simulink library "PalmaLibs"  (Simulink 8.1)
settings: Solver=ode45  SolverMode=SingleTasking  StartTime=0.0  StopTime=10.0  RelTol=1e-3
undefined symbols (not defined in the file or in its folder): gca, lambda1, lambda2, playNice, pls_solve, w_0
undefined symbols (not defined in the file): beta, w, Xpost, Xpre
libraries: simulink x9, dspmtrx3 x2, gated_decay_choice x2, range_choice x2, synaptic_scaling_choice x2, WaveformsLib x2, PalmaLibs x1, dspxfrm3 x1, CurrentsLib x1, SynapsesLib x1
settings Model: Creator=jpalma  LastModifiedBy=Leo

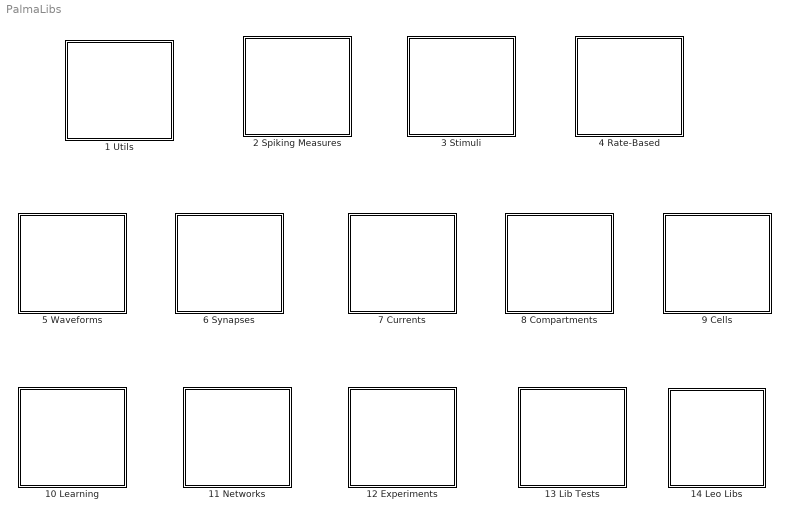
== system PalmaLibs ==
  " 1 Utils" : Subsystem
      mask help: Library Designer: Jesse Palma
      settings: OpenFcn=UtilsLib
      mask Help: Library Designer: Jesse Palma
      mask Display: image(imread('../Libs/icons/Utils.JPG'),'Center');
  " 2 Spiking Measures" : Subsystem
      mask help: Library Designer: Jesse Palma
      settings: OpenFcn=SpikingLib
      mask Help: Library Designer: Jesse Palma
      mask Display: image(imread('../Libs/icons/BasicSpike.JPG'),'Center')
  " 3 Stimuli" : Subsystem
      mask help: Library Designer: Jesse Palma
      settings: OpenFcn=StimuliLib
      mask Help: Library Designer: Jesse Palma
      mask Display: image(imread('../Libs/icons/Stimuli.JPG'),'Center')
  " 4 Rate-Based" : Subsystem
      mask help: Library Designer: Jesse Palma
      settings: OpenFcn=RateBasedLib
      mask Help: Library Designer: Jesse Palma
      mask Display: image(imread('../Libs/icons/RateBased.JPG'),'Center')
  " 5 Waveforms" : Subsystem
      mask help: Library Designer: Jesse Palma
      settings: OpenFcn=WaveformsLib
      mask Help: Library Designer: Jesse Palma
      mask Display: image(imread('../Libs/icons/DoubleExp.JPG'),'center');
  " 6 Synapses" : Subsystem
      mask help: Library Designer: Jesse Palma
      settings: OpenFcn=SynapsesLib
      mask Help: Library Designer: Jesse Palma
      mask Display: image(imread('../Libs/icons/Synapse.JPG'),'center');
  " 7 Currents" : Subsystem
      mask help: Library Designer: Jesse Palma
      settings: OpenFcn=CurrentsLib
      mask Help: Library Designer: Jesse Palma
      mask Display: image(imread('../Libs/icons/Channel.JPG'),'center');
  " 8 Compartments" : Subsystem
      mask help: Library Designer: Jesse Palma
      settings: OpenFcn=CompartmentsLib
      mask Help: Library Designer: Jesse Palma
      mask Display: image(imread('../Libs/icons/Compartment.JPG'),'Center')
  " 9 Cells" : Subsystem
      mask help: Library Designer: Jesse Palma
      settings: OpenFcn=CellsLib
      mask Help: Library Designer: Jesse Palma
      mask Display: image(imread('../Libs/icons/Cell.JPG'),'center');
  10 Learning : Subsystem
      mask help: Library Designer: Jesse Palma
      settings: OpenFcn=LearningLib
      mask Help: Library Designer: Jesse Palma
      mask Display: image(imread('../Libs/icons/Synapse.JPG'),'center');
  11 Networks : Subsystem
      mask help: Library Designer: Jesse Palma
      settings: OpenFcn=NetworksLib
      mask Help: Library Designer: Jesse Palma
      mask Display: image(imread('../Libs/icons/Networks.JPG'),'Center');
  12 Experiments : Subsystem
      mask help: Library Designer: Jesse Palma
      settings: OpenFcn=ExperimentsLib
      mask Help: Library Designer: Jesse Palma
      mask Display: image(imread('../Libs/icons/Experiments.JPG'),'Center');
  13 Lib Tests : Subsystem
      mask help: Library Designer: Jesse Palma
      settings: OpenFcn=LibTests
      mask Help: Library Designer: Jesse Palma
      mask Display: image(imread('../Libs/icons/LibTests.JPG'),'Center');
  14 Leo Libs : Subsystem

== system PalmaLibs/ 1 Utils ==

== system PalmaLibs/ 2 Spiking Measures ==

== system PalmaLibs/ 3 Stimuli ==

== system PalmaLibs/ 4 Rate-Based ==

== system PalmaLibs/ 5 Waveforms ==

== system PalmaLibs/ 6 Synapses ==

== system PalmaLibs/ 7 Currents ==

== system PalmaLibs/ 8 Compartments ==

== system PalmaLibs/ 9 Cells ==

== system PalmaLibs/10 Learning ==

== system PalmaLibs/11 Networks ==

== system PalmaLibs/12 Experiments ==

== system PalmaLibs/13 Lib Tests ==

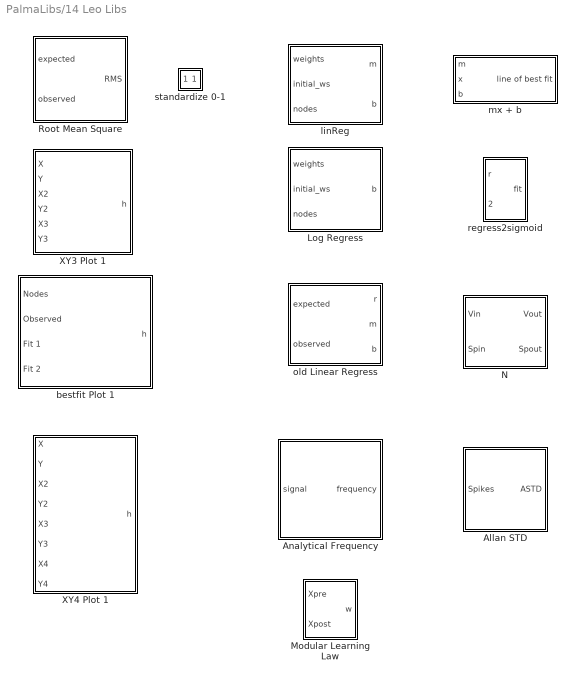
== system PalmaLibs/14 Leo Libs ==
  Allan STD : Subsystem  mask{tao=50}
      mask prompts: tao "time window"
  Analytical Frequency : Subsystem  mask{freqWindow=1}
      mask prompts: freqWindow "Window (time steps)"
      mask init:
      | freqWindow = 1;
      mask Display:
      | image(imread('../Libs/icons/hilbert.jpg'),'center');
      | port_label('input',1,'signal');
      | port_label('output',1,'freq');
  Log Regress : Subsystem  mask(Regression){numNodes=10}
      mask prompts: numNodes "Number of Nodes:"
      mask help:
      | This block does a nonlinear regression and returns the parameters necessary
      | for reconstruction
      mask init:
      | setupRegress(numNodes);
      mask Display:
      | image(imread('../Libs/icons/logfit.jpg'),'center');
      | port_label('input',1,'weights');
      | port_label('input',2,'initial weights');
      | port_label('input',3,'nodes');
      | port_label('output',1,'r');
  Modular Learning Law : Subsystem  mask{gorch_y_n=on, gated_decay=Dual OR, multdiv=Divide, synscale=Vanilla Oja, gorch_range=0, lambda1=1, lambda2=0, lambda3=0, lambda4=0, w_0=0, w0=0, alpha1=0, alpha2=0, beta=0, equ=lambda2*[Xpre*Xpost*(gorchrange)+ lambda1*(w_0-w) / ((alpha1*Xpre+alpha2*Xpost^2)*(w-w_0)) + .5lambda3*lambda4*(w_0 - w)comp(w_0,w)*(g(Xpost) - |g(Xpost)|)(g(Xpost))], extr=}
      mask prompts: gorch_y_n "Would you like a Gorch range?"; gated_decay "What kind of gated decay do you want"; multdiv "Multiply or Divide by the Gated Decay"; synscale "Synaptic Scaling"; gorch_range "Gorch Range"; lambda1 "Learning Rate (1) - Stability"; lambda2 "Learning Rate (2) - Total"; lambda3 "Learning Rate (3, Oja Specific) - Increment"; lambda4 "Learning Rate (4, Oja Specific) - Decrement"; w_0 "Range"; w0 "Initial weight"; alpha1 "Alpha 1 (Additional Parameter)"; alpha2 "Alpha 2 (Additional Parameter)"; beta "Beta (Gorch Gating Term)"; equ "Equation"; extr "Extra info"
      mask help: Make sure to hit apply after selecting your Law Type before moving on to the Law Parameters Tab.
      mask init:
      | eqw ='lambda2*[';
      | dab = gcb;
      | set_param(dab,'extr','');
      | currentVis = get_param(dab,'MaskVisibilities');
      | currentVis{12} = 'off';
      | currentVis{13} = 'off';
      | currentVis{14} = 'off';
      | 
      | if(gorch_y_n)
      |     set_param([dab '/Range'], 'BlockChoice', 'Gorch_range');
      |     currentVis{5} = 'on';
      |     eqw = [eqw 'Xpre*Xpost*(gorchrange)'];
      | else
      |     set_param([dab '/Range'], 'BlockChoice', 'Simple');
      |     currentVis{5} = 'off';
      |     eqw = [eqw 'Xpre*Xpost'];
      | end
      | 
      | eqw = [eqw '+ lambda1*(w_0-w)']
      | 
      | switch multdiv
      |     case 1 %'Multiply'
      |         set_param([dab '/TimesOrDivide'],'Inputs','**');
      |         eqw = [eqw ' * '];
      |     case 2 %'Divide'
      |         set_param([dab '/TimesOrDivide'],'Inputs','*/');
      |         eqw = [eqw ' / '];
      |     case 3 %'Inverse Divide'
      |         set_param([dab '/TimesOrDivide'],'Inputs','/*');
      |         eqw = [eqw ' \ '];
      | end
      | 
      | switch gated_decay
      |     case 1 %'Xpre'
      |         set_param([dab '/Gated Decay Choice'], 'BlockChoice', 'X_pre');
      |         eqw = [eqw 'Xpre'];
      |     case 2 %'Xpost'
      |         set_param([dab '/Gated Decay Choice'], 'BlockChoice', 'X_post');
      |         eqw = [eqw 'Xpost'];
      |     case 3 %'Gorch'
      |         set_param([dab '/Gated Decay Choice'], 'BlockChoice', 'Gorch_Gating');
      |         eqw = [eqw '(Xpost^2 * beta)'];
      |         currentVis{14} = 'on';
      |     case 4 %'Oja'
      |         set_param([dab '/Gated Decay Choice'], 'BlockChoice', 'Oja_Gating');
      |         eqw = [eqw '(Xpost^2*(w-w_0))'];
      |         currentVis{14} = 'off';
      |     case 5 %'Dual OR'
      |         set_param([dab '/Gated Decay Choice'], 'BlockChoice', 'Dual_OR');
      |         eqw = [eqw '((alpha1*Xpre+alpha2*Xpost^2)*(w-w_0))'];
      |         currentVis{12} = 'on';
      |         currentVis{13} = 'on';
      |     case 6 %'Dual AND'
      |         set_param([dab '/Gated Decay Choice'], 'BlockChoice', 'Dual_AND');
      |         eqw = [eqw '(alpha1*Xpre*Xpost^2*(w-w_0))'];
      |         currentVis{12} = 'on';
      | end
      | 
      | switch synscale
      |     case 1 %none
      |         set_param([dab '/Synaptic Scaling Choice'], 'BlockChoice', 'None');
      |         currentVis{8} = 'off';
      |         currentVis{9} = 'off';
      |         eqw = [eqw ']']
      |     case 2 %oja
      |         set_param([dab '/Synaptic Scaling Choice'], 'BlockChoice', 'Oja_stock');
      |         currentVis{8} = 'on';
      |         currentVis{9} = 'on';
      |         eqw = [eqw ' + .5lambda3*lambda4*(w_0 - w)comp(w_0,w)*(g(Xpost) - |g(Xpost)|)(g(Xpost))]'];
      |         set_param(dab,'extr','dg(X)/dt = s-AX, g(0) = -t, comp(w0,w) = |w0-w| <= range');
      | end
      | 
      | set_param(dab,'MaskVisibilities',currentVis);
      | set_param(dab,'equ',eqw);
      settings: AttributesFormatString=dw/dt = %<equ>\n%<extr>
      mask TypeOptions gated_decay: Xpre | Xpost | Gorch | Oja | Dual OR | Dual AND
      mask TypeOptions multdiv: Multiply | Divide | Inverse Divide
      mask TypeOptions synscale: None | Vanilla Oja
  N : Subsystem
  Root Mean Square : Subsystem  mask(Root Mean Square){}
      mask help: This block returns the root mean square error associated with an expected value and an observed value
      mask Display:
      | image(imread('../Libs/icons/rms.jpg'),'center');
      | port_label('input',1,'Expected');
      | port_label('input',2,'Observed');
      | port_label('output',1,'RMS');
  XY3 Plot 1 : Subsystem  AncestorBlock=UtilsLib/XY3 Plot  mask{plotInt=10, plotFig=1}
      mask prompts: plotInt "Plotting Interval (Sim steps)"; plotFig "Figure Number"
      mask help: The number of the block is the number of the figure
      mask init:
      | temp = get_param(gcb, 'Name');
      | plotFig = findLastNums(temp);
      mask Display: image(imread('../Libs/icons/XYFunc.JPG'),'center');
  XY4 Plot 1 : Subsystem  AncestorBlock=PalmaLibs/14 Leo Libs/XY3 Plot 1  mask{plotInt=10, plotFig=1}
      mask prompts: plotInt "Plotting Interval (Sim steps)"; plotFig "Figure Number"
      mask help: The number of the block is the number of the figure
      mask init:
      | temp = get_param(gcb, 'Name');
      | plotFig = findLastNums(temp);
      mask Display: image(imread('../Libs/icons/XYFunc.JPG'),'center');
  bestfit Plot 1 : Subsystem  AncestorBlock=PalmaLibs/14 Leo Libs/XY3 Plot 1  mask{plotInt=10, plotFig=1}
      mask prompts: plotInt "Plotting Interval (Sim steps)"; plotFig "Figure Number"
      mask help: The number of the block is the number of the figure
      mask init:
      | temp = get_param(gcb, 'Name');
      | plotFig = findLastNums(temp);
      mask Display: image(imread('../Libs/icons/XYFunc.JPG'),'center');
  linReg : Subsystem  mask{numNodes=10}
      mask prompts: numNodes "Number of Nodes"
      mask init:
      | setupLinRegress(numNodes)
      mask Display:
      | image(imread('../Libs/icons/regressionsweb.jpg'),'center');
      | port_label('input',1,'Weights');
      | port_label('input',2,'ws0');
      | port_label('input',3,'Nodes');
      | port_label('output',1,'m');
      | port_label('output',2,'b');
  mx + b : Subsystem
      mask help: Helper block for linReg, takes fitted params and produces the associated line
  old Linear Regress : Subsystem  mask(Regression){}
      mask help:
      | This block does a linear regression between expected and observed data in blocks of 100 trials.
      | Returns r,m,b values of regression
      mask Display:
      | image(imread('../Libs/icons/regressionsweb.jpg'),'center');
      | port_label('input',1,'Expected');
      | port_label('input',2,'Observed');
      | port_label('output',1,'r');
      | port_label('output',2,'m');
      | port_label('output',3,'b');
  regress2sigmoid : Subsystem
      mask help: Helper block for logRegress, takes fitted params and produces the associated curve
  standardize 0-1 : Subsystem
      mask help: Standardize input to range 0-1

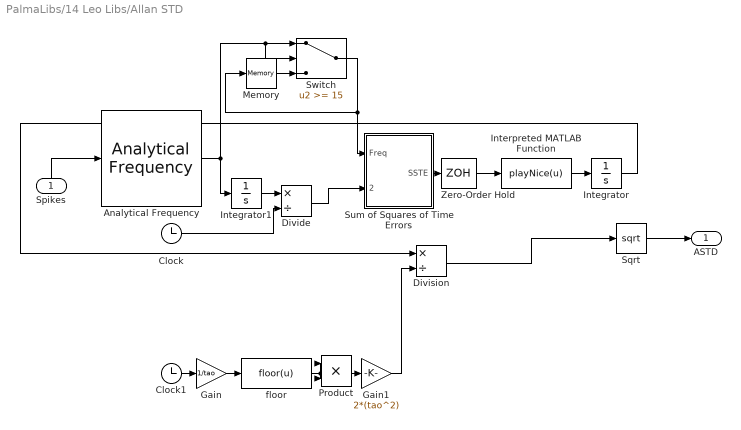
== system PalmaLibs/14 Leo Libs/Allan STD ==
  Spikes : Inport
  Analytical Frequency : PalmaLibs/14 Leo Libs/Analytical Frequency  freqWindow=1
  Clock : Clock
  Clock1 : Clock
  Divide : Product  Inputs=*/
  Division : Product  Inputs=*/
  Gain : Gain  Gain=1/tao
  Gain1 : Gain  Gain=2*(tao^2)
  Integrator : Integrator
  Integrator1 : Integrator
  Interpreted MATLAB Function : MATLABFcn  MATLABFcn=playNice(u)
  Memory : Memory
  Product : Product
  Sqrt : Sqrt  SaturateOnIntegerOverflow=on
  Sum of Squares of Time Errors : Subsystem
  Switch : Switch  Threshold=15
  Zero-Order Hold : ZeroOrderHold  SampleTime=tao
  floor : MATLABFcn  MATLABFcn=floor(u)
  ASTD : Outport
  wires:
  Sum of Squares of Time Errors/1(SSTE) -> Zero-Order Hold/1
  Clock1/1 -> Gain/1
  Gain/1 -> floor/1
  floor/1 -> Product/2, Product/1
  Product/1 -> Gain1/1
  Gain1/1 -> Division/2
  Division/1 -> Sqrt/1
  Sqrt/1 -> ASTD/1
  Integrator/1 -> Division/1
  Zero-Order Hold/1 -> Interpreted MATLAB Function/1
  Interpreted MATLAB Function/1 -> Integrator/1
  Spikes/1 -> Analytical Frequency/1
  Divide/1 -> Sum of Squares of Time Errors/2(nomFreq)
  Analytical Frequency/1 -> Switch/2, Switch/1, Integrator1/1
  Integrator1/1 -> Divide/1
  Clock/1 -> Divide/2
  Switch/1 -> Sum of Squares of Time Errors/1(Freq), Memory/1
  Memory/1 -> Switch/3

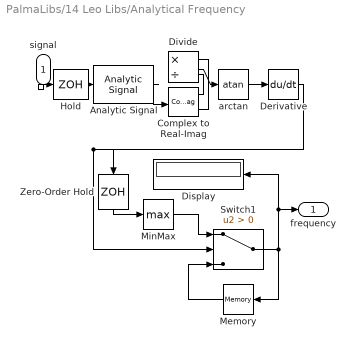
== system PalmaLibs/14 Leo Libs/Analytical Frequency ==
  signal : Inport
  Analytic Signal : dspxfrm3/Analytic Signal  N=100  InputProcessing=Columns as channels (frame based)
  Complex to Real-Imag : ComplexToRealImag
  Derivative : Derivative
  Display : Display
  Divide : Product  Inputs=*/
  Hold : ZeroOrderHold
  Memory : Memory
  MinMax : MinMax  Function=max
  Switch1 : Switch  Criteria=u2 > Threshold
  Zero-Order Hold : ZeroOrderHold  SampleTime=freqWindow
  arctan : Trigonometry  Operator=atan
  frequency : Outport
  wires:
  arctan/1 -> Derivative/1
  Divide/1 -> arctan/1
  Complex to Real-Imag/2 -> Divide/1
  Complex to Real-Imag/1 -> Divide/2
  Analytic Signal/1 -> Complex to Real-Imag/1
  Memory/1 -> Switch1/3
  Switch1/1 -> frequency/1, Display/1, Memory/1
  Zero-Order Hold/1 -> MinMax/1
  Derivative/1 -> Switch1/2, Zero-Order Hold/1
  MinMax/1 -> Switch1/1
  signal/1 -> Hold/1
  Hold/1 -> Analytic Signal/1

== system PalmaLibs/14 Leo Libs/Log Regress ==
  weights : Inport
  initial_ws : Inport  Port=2
  nodes : Inport  Port=3
  Compare To Constant : simulink/Logic and Bit Operations/Compare To Constant  relop=<=  const=Inf  OutDataTypeStr=uint8
  Hold1 : ZeroOrderHold  SampleTime=100
  Hold2 : ZeroOrderHold  SampleTime=100
  Hold3 : ZeroOrderHold  SampleTime=100
  Switch : Switch  Threshold=1
  Transpose : dspmtrx3/Transpose  Hermitian=off  overflowFlag=off
  Vector Concatenate : Concatenate
  solver : MATLABFcn  MATLABFcn=pls_solve([u(11),u(12),u(13),u(14),u(15),u(16),u(17),u(18),u(19),u(20)],[u(1),u(2),u(3),u(4),u(5),u(6),u(7),u(8),u(9),u(10)],[ 0.1 0 0.1])
  b : Outport
  wires:
  Hold3/1 -> Vector Concatenate/2
  Hold2/1 -> Switch/3
  Vector Concatenate/1 -> solver/1
  nodes/1 -> Hold3/1
  initial_ws/1 -> Hold2/1
  Switch/1 -> Vector Concatenate/1
  Compare To Constant/1 -> Switch/2
  Transpose/1 -> Switch/1, Compare To Constant/1
  Hold1/1 -> Transpose/1
  weights/1 -> Hold1/1
  solver/1 -> b/1

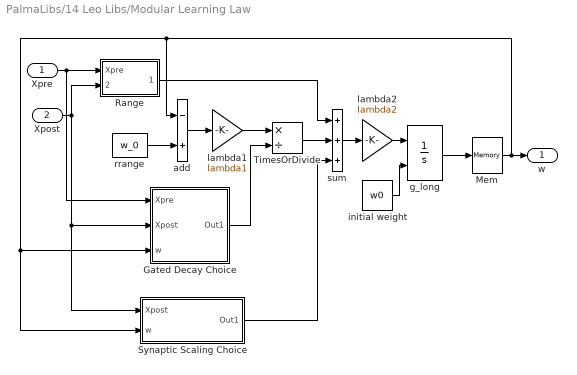
== system PalmaLibs/14 Leo Libs/Modular Learning Law ==
  Xpre : Inport
  Xpost : Inport  Port=2
  Gated Decay Choice : Subsystem  BlockChoice=Dual_OR
      settings: AttributesFormatString=%<BlockChoice>  TemplateBlock=gated_decay_choice/Gated Decay Choice  MemberBlocks=Dual_AND,Dual_OR,Gorch_Gating,Oja_Gating,X_post,X_pre
  Mem : Memory
  Range : Subsystem  BlockChoice=Gorch_range
      link override Gorch_range/range: Value=gorch_range
      settings: AttributesFormatString=%<BlockChoice>  TemplateBlock=range_choice/Range  MemberBlocks=Gorch_range,Simple
  Synaptic Scaling Choice : Subsystem  BlockChoice=Oja_stock
      settings: AttributesFormatString=%<BlockChoice>  TemplateBlock=synaptic_scaling_choice/Synaptic Scaling Choice  MemberBlocks=None,Oja_stock
  TimesOrDivide : Product  Inputs=*/
  add : Sum  Inputs=-+
  g_long : Integrator  InitialConditionSource=external  ZeroCross=off
  initial weight : Constant  Value=w0
  lambda1 : Gain  Gain=lambda1
  lambda2 : Gain  Gain=lambda2
  rrange : Constant  Value=w_0
  sum : Sum  Inputs=+++
  w : Outport
  wires:
  Xpre/1 -> Range/1(Xpre), Gated Decay Choice/1(Xpre)
  Xpost/1 -> Gated Decay Choice/2(Xpost), Synaptic Scaling Choice/1(Xpost), Range/2(Xpost)
  rrange/1 -> add/2
  Range/1(Out1) -> sum/1
  add/1 -> lambda1/1
  lambda1/1 -> TimesOrDivide/1
  TimesOrDivide/1 -> sum/2
  g_long/1 -> Mem/1
  initial weight/1 -> g_long/2
  Mem/1 -> Synaptic Scaling Choice/2(w), Gated Decay Choice/3(w), add/1, w/1
  Gated Decay Choice/1(Out1) -> TimesOrDivide/2
  lambda2/1 -> g_long/1
  sum/1 -> lambda2/1
  Synaptic Scaling Choice/1(Out1) -> sum/3

== system PalmaLibs/14 Leo Libs/N ==
  Vin : Inport
  Spin : Inport  Port=2
  AMPASynapse : Subsystem  AncestorBlock=SynapsesLib/CompoundDiffSynapse  mask{EZ=0, gZ=0.05, tauRZ=1, tauFZ=6}
      mask prompts: EZ "Eq Voltage, EZ"; gZ "Conductance, gZ"; tauRZ "Rise Time, tauRZ"; tauFZ "Fall Time, tauFZ"
      mask help: Author: Jesse Palma
      mask Help: Author: Jesse Palma
      mask Display: image(imread('../Libs/icons/Synapse.jpg'),'center');
  Add : Sum
  Izhikevich Book1 : Subsystem  AncestorBlock=CompartmentsLib/Izhikevich Book  mask{settings=UserDefined, A=0.03, B=-2, C=-50, D=100, CP=100, K=0.7, VR=-60, VT=-40, VP=35, V0=-60, U0=0}
      mask prompts: settings "Parameter Settings"; A "a, recovery u time constant"; B "b, dynamics parameter"; C "c,  reset value v"; D "d, reset shift u"; CP "Cp, capacitance"; VR "Vr, voltage rest"; VT "Vt, voltage threshold"; VP "Vpeak, voltage peak reset"; V0 "V0, initial v value"; U0 "U0, initial u value"
      mask help:
      | Model from Eugene Izhikevich's book "Dynamical Systems in Neuroscience"
      |     (Equations 8.5 & 8.6 on page 273)
      | 9 Paramters are reducable to 4-parameter model.
      |
      | Simulink Model Design: Jesse Palma
      mask Help:
      | Model from Eugene Izhikevich's book
      | <a href=http://www.izhikevich.org/publications/dsn/index.htm>"Dynamical Systems in Neuroscience"</a>
      | <br>(Equations 8.5 & 8.6 on page 273)<br>
      | 9 Paramters are reducable to 4-parameter model.
      | <br><br>
      | Simulink Model Design: Jesse Palma
      mask TypeOptions settings: Regular-Spiking(p274-283) | Motor(p287) | UserDefined
      mask Callback settings:
      | maskStr = get_param(gcb,'MaskValues');
      | if strcmp(maskStr{1},'Regular-Spiking(p274-283)')
      |    maskStr = get_param(gcb,'MaskValues');
      |    maskStr{2} = '0.03'; %A
      |    maskStr{3} = '-2';   %B
      |    maskStr{4} = '-50';  %C
      |    maskStr{5} = '100';  %D
      |    maskStr{6} = '100';  %CP
      |    maskStr{7} = '0.7';  %K
      |    maskStr{8} = '-60';  %VR
      |    maskStr{9} = '-40';  %VT
      |    maskStr{10} = '35';  %VP
      |    maskStr{11} = '-60'; %V0
      |    maskStr{12} = '0';   %U0
      |    set_param(gcb, 'MaskValues', maskStr);
      | end
      | if strcmp(maskStr{1},'Motor(p287)')
      |    maskStr = get_param(gcb,'MaskValues');
      |    maskStr{2} = '0.01'; %A
      |    maskStr{3} = '-0.25';%B
      |    maskStr{4} = '-40';  %C
      |    maskStr{5} = '90';   %D
      |    maskStr{6} = '30';   %CP
      |    maskStr{7} = '3';    %K
      |    maskStr{8} = '-55';  %VR
      |    maskStr{9} = '-42';  %VT
      |    maskStr{10} = '10';  %VP
      |    maskStr{11} = '-55'; %V0
      |    maskStr{12} = '0';   %U0
      |    set_param(gcb, 'MaskValues', maskStr);
      | end
      mask Callback A:
      | maskStr = get_param(gcb,'MaskValues');
      | maskStr{1} = 'UserDefined';
      | set_param(gcb, 'MaskValues', maskStr);
      mask Callback B:
      | maskStr = get_param(gcb,'MaskValues');
      | maskStr{1} = 'UserDefined';
      | set_param(gcb, 'MaskValues', maskStr);
      mask Callback C:
      | maskStr = get_param(gcb,'MaskValues');
      | maskStr{1} = 'UserDefined';
      | set_param(gcb, 'MaskValues', maskStr);
      mask Callback D:
      | maskStr = get_param(gcb,'MaskValues');
      | maskStr{1} = 'UserDefined';
      | set_param(gcb, 'MaskValues', maskStr);
      mask Callback CP:
      | maskStr = get_param(gcb,'MaskValues');
      | maskStr{1} = 'UserDefined';
      | set_param(gcb, 'MaskValues', maskStr);
      mask Callback K:
      | maskStr = get_param(gcb,'MaskValues');
      | maskStr{1} = 'UserDefined';
      | set_param(gcb, 'MaskValues', maskStr);
      mask Callback VR:
      | maskStr = get_param(gcb,'MaskValues');
      | maskStr{1} = 'UserDefined';
      | set_param(gcb, 'MaskValues', maskStr);
      mask Callback VT:
      | maskStr = get_param(gcb,'MaskValues');
      | maskStr{1} = 'UserDefined';
      | set_param(gcb, 'MaskValues', maskStr);
      mask Callback VP:
      | maskStr = get_param(gcb,'MaskValues');
      | maskStr{1} = 'UserDefined';
      | set_param(gcb, 'MaskValues', maskStr);
      mask Callback V0:
      | maskStr = get_param(gcb,'MaskValues');
      | maskStr{1} = 'UserDefined';
      | set_param(gcb, 'MaskValues', maskStr);
      mask Callback U0:
      | maskStr = get_param(gcb,'MaskValues');
      | maskStr{1} = 'UserDefined';
      | set_param(gcb, 'MaskValues', maskStr);
      mask Display: image(imread('../Libs/icons/Izhik.jpg'),'center');
  Learning Law : Subsystem  mask{gorch_y_n=off, gated_decay=Gorch, multdiv=Multiply, synscale=None, gorch_range=0, lambda1=.05, lambda2=.05, lambda3=0, lambda4=0, w_0=1, w0=.3, beta=1, equ=lambda2*[Xpre*Xpost+ lambda1*(w_0-w) * (Xpost^2 * beta)], extr=}
      mask prompts: gorch_y_n "Would you like a Gorch range?"; gated_decay "What kind of gated decay do you want"; multdiv "Multiply or Divide by the Gated Decay"; synscale "Synaptic Scaling"; gorch_range "Gorch Range"; lambda1 "Learning Rate (1) - Stability"; lambda2 "Learning Rate (2) - Total"; lambda3 "Learning Rate (3, Oja Specific) - Increment"; lambda4 "Learning Rate (4, Oja Specific) - Decrement"; w_0 "Range"; w0 "Initial weight"; beta "Beta (Gorch Gating Term)"; equ "Equation"; extr "Extra info"
      mask help: Make sure to hit apply after selecting your Law Type before moving on to the Law Parameters Tab.
      mask init:
      | eqw ='lambda2*[';
      | dab = gcb;
      | set_param(dab,'extr','');
      | currentVis = get_param(dab,'MaskVisibilities');
      | if(gorch_y_n)
      |     set_param([dab '/Range'], 'BlockChoice', 'Gorch_range');
      |     currentVis{5} = 'on';
      |     eqw = [eqw 'Xpre*Xpost*(gorchrange)'];
      | else
      |     set_param([dab '/Range'], 'BlockChoice', 'Simple');
      |     currentVis{5} = 'off';
      |     currentVis{12} = 'off';
      |     eqw = [eqw 'Xpre*Xpost'];
      | end
      | eqw = [eqw '+ lambda1*(w_0-w)']
      | switch multdiv
      |     case 1 %'Multiply'
      |         set_param([dab '/TimesOrDivide'],'Inputs','**');
      |         eqw = [eqw ' * '];
      |     case 2 %'Divide'
      |         set_param([dab '/TimesOrDivide'],'Inputs','*/');
      |         eqw = [eqw ' / '];
      |         
      |     case 3 %'Inverse Divide'
      |         set_param([dab '/TimesOrDivide'],'Inputs','/*');
      |         eqw = [eqw ' \ '];
      |         
      | end
      | switch gated_decay
      |     case 1 %'Xpre'
      |         set_param([dab '/Gated Decay Choice'], 'BlockChoice', 'X_pre');
      |         eqw = [eqw 'Xpre'];
      |         currentVis{12} = 'off';
      |         
      |     case 2 %'Xpost'
      |         set_param([dab '/Gated Decay Choice'], 'BlockChoice', 'X_post');
      |         eqw = [eqw 'Xpost'];
      |         currentVis{12} = 'off';
      |         
      |     case 3 %'Gorch'
      |         set_param([dab '/Gated Decay Choice'], 'BlockChoice', 'Gorch_Gating');
      |         eqw = [eqw '(Xpost^2 * beta)'];
      |         currentVis{12} = 'on';
      |         
      |     case 4 %'Oja'
      |         set_param([dab '/Gated Decay Choice'], 'BlockChoice', 'Oja_Gating');
      |         eqw = [eqw '(Xpost^2*(w-w_0))'];
      |         currentVis{12} = 'off';
      |         
      | end
      | 
      | switch synscale
      |     case 1 %none
      |         set_param([dab '/Synaptic Scaling Choice'], 'BlockChoice', 'None');
      |         currentVis{8} = 'off';
      |         currentVis{9} = 'off';
      |         eqw = [eqw ']']
      |     case 2 %oja
      |         set_param([dab '/Synaptic Scaling Choice'], 'BlockChoice', 'Oja_stock');
      |         currentVis{8} = 'on';
      |         currentVis{9} = 'on';
      |         eqw = [eqw ' + .5lambda3*lambda4*(w_0 - w)comp(w_0,w)*(g(Xpost) - |g(Xpost)|)(g(Xpost))]'];
      |         set_param(dab,'extr','dg(X)/dt = s-AX, g(0) = -t, comp(w0,w) = |w0-w| <= range');
      | end
      | set_param(dab,'MaskVisibilities',currentVis);
      | set_param(dab,'equ',eqw);
      settings: AttributesFormatString=dw/dt = %<equ>\n%<extr>
      mask TypeOptions gated_decay: Xpre | Xpost | Gorch | Oja
      mask TypeOptions multdiv: Multiply | Divide | Inverse Divide
      mask TypeOptions synscale: None | Vanilla Oja
  Memory : Memory  X0=0.3
  NMDASynapse1 : SynapsesLib/NMDASynapse  EZ=0  gZ=0.005  tauRZ=0.33  tauFZ=40  etaZ=0.33  mgZ=1  gammaZ=0.06  gainZ=4
  Spike Simpl : WaveformsLib/Spike Simpl  a=-0.2  b=0.65  c=0.05
  gain1 : Gain  Gain=45
  Vout : Outport
  Spout : Outport  Port=2
  wires:
  Spin/1 -> Learning Law/1(Xpre), NMDASynapse1/1, AMPASynapse/1(spike_i)
  Vin/1 -> AMPASynapse/3(postv_j), NMDASynapse1/3
  gain1/1 -> Izhikevich Book1/1(I)
  Add/1 -> gain1/1
  NMDASynapse1/3 -> Add/1
  AMPASynapse/3(I) -> Add/2
  Izhikevich Book1/3(sp) -> Spike Simpl/2
  Izhikevich Book1/1(v) -> Vout/1, Spike Simpl/1
  Spike Simpl/1 -> Learning Law/2(Xpost), Spout/1
  Learning Law/1(w) -> Memory/1
  Memory/1 -> NMDASynapse1/2, AMPASynapse/2(w_ij)

== system PalmaLibs/14 Leo Libs/Root Mean Square ==
  expected : Inport
  observed : Inport  Port=2
  Gain : Gain  Gain=.5
  Hold : ZeroOrderHold  SampleTime=100
  Hold1 : ZeroOrderHold  SampleTime=100
  Sqrt : Sqrt  SaturateOnIntegerOverflow=on
  Sum : Sum  Inputs=|+-
  square : Math  Operator=square  SaturateOnIntegerOverflow=on
  RMS : Outport
  wires:
  expected/1 -> Hold/1
  observed/1 -> Hold1/1
  Hold1/1 -> Sum/2
  Hold/1 -> Sum/1
  Sum/1 -> square/1
  Gain/1 -> Sqrt/1
  Sqrt/1 -> RMS/1
  square/1 -> Gain/1

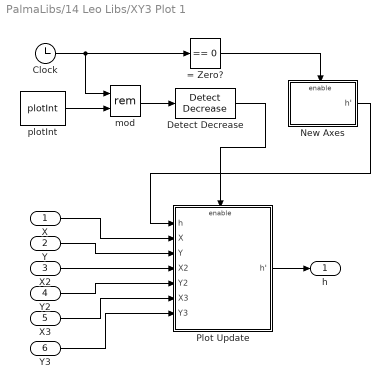
== system PalmaLibs/14 Leo Libs/XY3 Plot 1 ==
  X : Inport
  Y : Inport  Port=2
  X2 : Inport  Port=3
  Y2 : Inport  Port=4
  X3 : Inport  Port=5
  Y3 : Inport  Port=6
  = Zero? : simulink/Logic and Bit Operations/Compare To Zero  relop===  OutDataTypeStr=uint8
  Clock : Clock
  Detect Decrease : simulink/Logic and Bit Operations/Detect Decrease  vinit=0.0  InputProcessing=Inherited  OutDataTypeStr=uint8
  New Axes : Subsystem
  Plot Update : Subsystem
  mod : Math  Operator=rem  SaturateOnIntegerOverflow=on
  plotInt : Constant  Value=plotInt
  h : Outport
  wires:
  Y2/1 -> Plot Update/5(Y2)
  X2/1 -> Plot Update/4(X2)
  X/1 -> Plot Update/2(X)
  Plot Update/1(h') -> h/1
  Y/1 -> Plot Update/3(Y)
  plotInt/1 -> mod/2
  Clock/1 -> mod/1, = Zero?/1
  mod/1 -> Detect Decrease/1
  = Zero?/1 -> New Axes/Enable
  Detect Decrease/1 -> Plot Update/Enable
  New Axes/1(h') -> Plot Update/1(h)
  X3/1 -> Plot Update/6(X3)
  Y3/1 -> Plot Update/7(Y3)

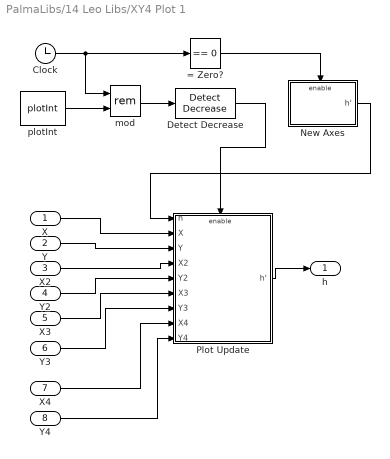
== system PalmaLibs/14 Leo Libs/XY4 Plot 1 ==
  X : Inport
  Y : Inport  Port=2
  X2 : Inport  Port=3
  Y2 : Inport  Port=4
  X3 : Inport  Port=5
  Y3 : Inport  Port=6
  X4 : Inport  Port=7
  Y4 : Inport  Port=8
  = Zero? : simulink/Logic and Bit Operations/Compare To Zero  relop===  OutDataTypeStr=uint8
  Clock : Clock
  Detect Decrease : simulink/Logic and Bit Operations/Detect Decrease  vinit=0.0  InputProcessing=Inherited  OutDataTypeStr=uint8
  New Axes : Subsystem
  Plot Update : Subsystem
  mod : Math  Operator=rem  SaturateOnIntegerOverflow=on
  plotInt : Constant  Value=plotInt
  h : Outport
  wires:
  Y3/1 -> Plot Update/7(Y3)
  X3/1 -> Plot Update/6(X3)
  New Axes/1(h') -> Plot Update/1(h)
  Detect Decrease/1 -> Plot Update/Enable
  = Zero?/1 -> New Axes/Enable
  mod/1 -> Detect Decrease/1
  Clock/1 -> = Zero?/1, mod/1
  plotInt/1 -> mod/2
  Y/1 -> Plot Update/3(Y)
  Plot Update/1(h') -> h/1
  X/1 -> Plot Update/2(X)
  X2/1 -> Plot Update/4(X2)
  Y2/1 -> Plot Update/5(Y2)
  X4/1 -> Plot Update/8(X4)
  Y4/1 -> Plot Update/9(Y4)

== system PalmaLibs/14 Leo Libs/bestfit Plot 1 ==
  Nodes : Inport
  Observed : Inport  Port=2
  Fit 1 : Inport  Port=3
  Fit 2 : Inport  Port=4
  = Zero? : simulink/Logic and Bit Operations/Compare To Zero  relop===  OutDataTypeStr=uint8
  Clock : Clock
  Detect Decrease : simulink/Logic and Bit Operations/Detect Decrease  vinit=0.0  InputProcessing=Inherited  OutDataTypeStr=uint8
  New Axes : Subsystem
  Plot Update : Subsystem
  mod : Math  Operator=rem  SaturateOnIntegerOverflow=on
  plotInt : Constant  Value=plotInt
  h : Outport
  wires:
  Fit 1/1 -> Plot Update/5(Y2)
  Nodes/1 -> Plot Update/2(X), Plot Update/4(X2), Plot Update/6(X3)
  Plot Update/1(h') -> h/1
  Observed/1 -> Plot Update/3(Y)
  plotInt/1 -> mod/2
  Clock/1 -> mod/1, = Zero?/1
  mod/1 -> Detect Decrease/1
  = Zero?/1 -> New Axes/Enable
  Detect Decrease/1 -> Plot Update/Enable
  New Axes/1(h') -> Plot Update/1(h)
  Fit 2/1 -> Plot Update/7(Y3)

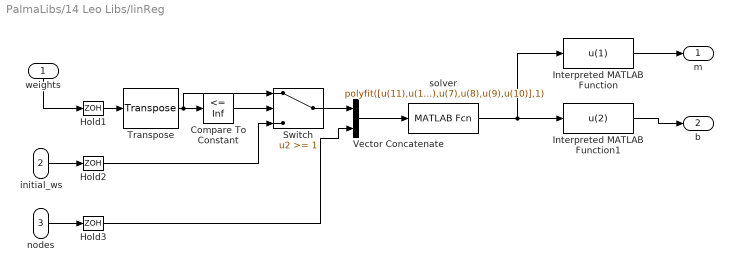
== system PalmaLibs/14 Leo Libs/linReg ==
  weights : Inport
  initial_ws : Inport  Port=2
  nodes : Inport  Port=3
  Compare To Constant : simulink/Logic and Bit Operations/Compare To Constant  relop=<=  const=Inf  OutDataTypeStr=uint8
  Hold1 : ZeroOrderHold  SampleTime=100
  Hold2 : ZeroOrderHold  SampleTime=100
  Hold3 : ZeroOrderHold  SampleTime=100
  Interpreted MATLAB Function : MATLABFcn  MATLABFcn=u(1)
  Interpreted MATLAB Function1 : MATLABFcn  MATLABFcn=u(2)
  Switch : Switch  Threshold=1
  Transpose : dspmtrx3/Transpose  Hermitian=off  overflowFlag=off
  Vector Concatenate : Concatenate
  solver : MATLABFcn  MATLABFcn=polyfit([u(11),u(12),u(13),u(14),u(15),u(16),u(17),u(18),u(19),u(20)],[u(1),u(2),u(3),u(4),u(5),u(6),u(7),u(8),u(9),u(10)],1)  mask{numNodes=0}
      mask prompts: numNodes "Number of Nodes"
      mask init:
      | %setupLinRegress(numNodes);
  m : Outport
  b : Outport  Port=2
  wires:
  Hold2/1 -> Switch/3
  Hold3/1 -> Vector Concatenate/2
  Hold1/1 -> Transpose/1
  Vector Concatenate/1 -> solver/1
  weights/1 -> Hold1/1
  Transpose/1 -> Compare To Constant/1, Switch/1
  Compare To Constant/1 -> Switch/2
  Switch/1 -> Vector Concatenate/1
  initial_ws/1 -> Hold2/1
  nodes/1 -> Hold3/1
  solver/1 -> Interpreted MATLAB Function/1, Interpreted MATLAB Function1/1
  Interpreted MATLAB Function/1 -> m/1
  Interpreted MATLAB Function1/1 -> b/1

== system PalmaLibs/14 Leo Libs/mx + b ==
  note: mx + b
  m : Inport
  x : Inport  Port=2
  b : Inport  Port=3
  Product1 : Product  RndMeth=Zero
  Sum1 : Sum  Inputs=|++
  line of best fit : Outport
  wires:
  Product1/1 -> Sum1/1
  Sum1/1 -> line of best fit/1
  m/1 -> Product1/1
  x/1 -> Product1/2
  b/1 -> Sum1/2

== system PalmaLibs/14 Leo Libs/old Linear Regress ==
  expected : Inport
  observed : Inport  Port=2
  Hold : ZeroOrderHold  SampleTime=100
  Hold1 : ZeroOrderHold  SampleTime=100
  regress b : M-S-Function  FunctionName=regress_block3
  regress m : M-S-Function  FunctionName=regress_block2
  regress r : M-S-Function  FunctionName=regress_block
  r : Outport
  m : Outport  Port=2
  b : Outport  Port=3
  wires:
  regress r/1 -> r/1
  regress m/1 -> m/1
  regress b/1 -> b/1
  observed/1 -> Hold1/1
  Hold1/1 -> regress r/2, regress m/2, regress b/2
  expected/1 -> Hold/1
  Hold/1 -> regress r/1, regress m/1, regress b/1

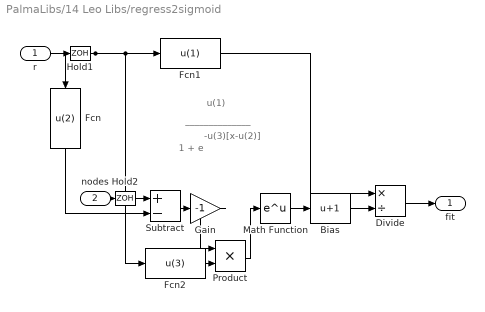
== system PalmaLibs/14 Leo Libs/regress2sigmoid ==
  note: ______________
  note: u(1)
  note: 1 + e
  note: -u(3)[x-u(2)]
  r : Inport
  nodes : Inport  Port=2
  Bias : Bias  Bias=1
  Divide : Product  Inputs=*/
  Fcn : Fcn  Expr=u(2)
  Fcn1 : Fcn  Expr=u(1)
  Fcn2 : Fcn  Expr=u(3)
  Gain : Gain  Gain=-1
  Hold1 : ZeroOrderHold  SampleTime=100
  Hold2 : ZeroOrderHold  SampleTime=100
  Math Function : Math  SaturateOnIntegerOverflow=on
  Product : Product  RndMeth=Zero
  Subtract : Sum  Inputs=+-
  fit : Outport
  wires:
  r/1 -> Hold1/1
  Fcn1/1 -> Divide/1
  Fcn/1 -> Subtract/2
  Math Function/1 -> Bias/1
  Bias/1 -> Divide/2
  nodes/1 -> Hold2/1
  Subtract/1 -> Gain/1
  Gain/1 -> Product/1
  Divide/1 -> fit/1
  Hold1/1 -> Fcn1/1, Fcn2/1, Fcn/1
  Hold2/1 -> Subtract/1
  Fcn2/1 -> Product/2
  Product/1 -> Math Function/1

== system PalmaLibs/14 Leo Libs/standardize 0-1 ==
  note: input will be time saturated data,
      | so i'll only normalize however much
      | there is for a certain interval for the
      | regression to work through
  note: Standardize X to range 0-1:
  Xi : Inport
  Divide : Product  Inputs=*/
  MinMax : MinMax
  MinMax1 : MinMax  Function=max
  Subtract : Sum  Inputs=+-
  Subtract1 : Sum  Inputs=-+
  Zero-Order Hold : ZeroOrderHold  SampleTime=100
  Si : Outport
  wires:
  Xi/1 -> Zero-Order Hold/1, Subtract/1
  Zero-Order Hold/1 -> MinMax/1, MinMax1/1
  Subtract/1 -> Divide/1
  Divide/1 -> Si/1
  MinMax/1 -> Subtract/2, Subtract1/1
  MinMax1/1 -> Subtract1/2
  Subtract1/1 -> Divide/2

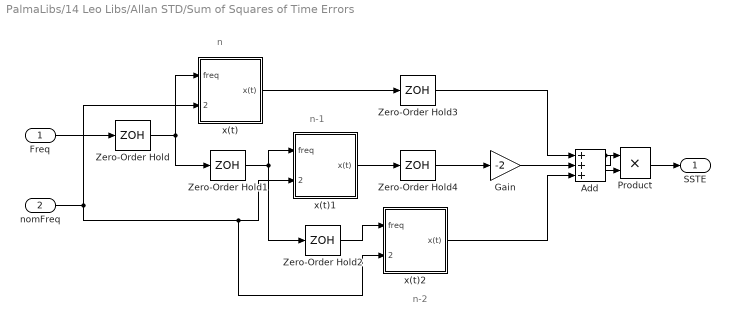
== system PalmaLibs/14 Leo Libs/Allan STD/Sum of Squares of Time Errors ==
  note: n
  note: n-2
  note: n-1
  Freq : Inport
  nomFreq : Inport  Port=2
  Add : Sum  Inputs=+++
  Gain : Gain  Gain=-2
  Product : Product
  Zero-Order Hold{,1..2,4} (4 alike) : ZeroOrderHold  SampleTime=tao
  Zero-Order Hold3 : ZeroOrderHold  SampleTime=2*tao
  x(t) : Subsystem
  x(t)1 : Subsystem
  x(t)2 : Subsystem
  SSTE : Outport
  wires:
  Gain/1 -> Add/2
  x(t)2/1(x(t)) -> Add/3
  Zero-Order Hold3/1 -> Add/1
  Zero-Order Hold4/1 -> Gain/1
  Add/1 -> Product/2, Product/1
  Zero-Order Hold1/1 -> x(t)1/1(freq), Zero-Order Hold2/1
  Zero-Order Hold/1 -> Zero-Order Hold1/1, x(t)/1(freq)
  x(t)/1(x(t)) -> Zero-Order Hold3/1
  x(t)1/1(x(t)) -> Zero-Order Hold4/1
  Zero-Order Hold2/1 -> x(t)2/1(freq)
  Freq/1 -> Zero-Order Hold/1
  Product/1 -> SSTE/1
  nomFreq/1 -> x(t)/2(nom_freq), x(t)2/2(nom_freq), x(t)1/2(nom_freq)

== system PalmaLibs/14 Leo Libs/Modular Learning Law/Gated Decay Choice ==
  Xpre : Inport
  Xpost : Inport  Port=2
  w : Inport  Port=3
  Dual_OR : gated_decay_choice/Dual_OR
  Out1 : Outport
  wires:
  Xpre/1 -> Dual_OR/1
  Xpost/1 -> Dual_OR/2
  w/1 -> Dual_OR/3
  Dual_OR/1 -> Out1/1

== system PalmaLibs/14 Leo Libs/Modular Learning Law/Range ==
  Xpre : Inport
  Xpost : Inport  Port=2
  Gorch_range : range_choice/Gorch_range
  Out1 : Outport
  wires:
  Xpre/1 -> Gorch_range/1
  Xpost/1 -> Gorch_range/2
  Gorch_range/1 -> Out1/1

== system PalmaLibs/14 Leo Libs/Modular Learning Law/Synaptic Scaling Choice ==
  Xpost : Inport
  w : Inport  Port=2
  Oja_stock : synaptic_scaling_choice/Oja_stock
  Out1 : Outport
  wires:
  Xpost/1 -> Oja_stock/1
  w/1 -> Oja_stock/2
  Oja_stock/1 -> Out1/1

== system PalmaLibs/14 Leo Libs/N/AMPASynapse ==
  spike_i : Inport
  w_ij : Inport  Port=2
  postv_j : Inport  Port=3
  Compound Diffentials : WaveformsLib/Compound Diffentials  tauRise=tauRZ  tauFall=tauFZ  squareWaveWidth=tauRZ  squareWaveHeight=1/tauRZ  interGain=2/tauRZ  finalGain=(tauFZ+tauRZ)/tauFZ
  Product : Product  RndMeth=Zero
  Sum_i : Product  Multiplication=Matrix(*)
  Ungated Current : CurrentsLib/Ungated Current  EX=EZ  gX=gZ
  T : Outport
  g : Outport  Port=2
  I : Outport  Port=3
  wires:
  w_ij/1 -> Sum_i/1
  Compound Diffentials/2 -> Sum_i/2
  Sum_i/1 -> g/1, Product/1
  postv_j/1 -> Ungated Current/1
  Compound Diffentials/1 -> T/1
  Ungated Current/1 -> Product/2
  spike_i/1 -> Compound Diffentials/1
  Product/1 -> I/1

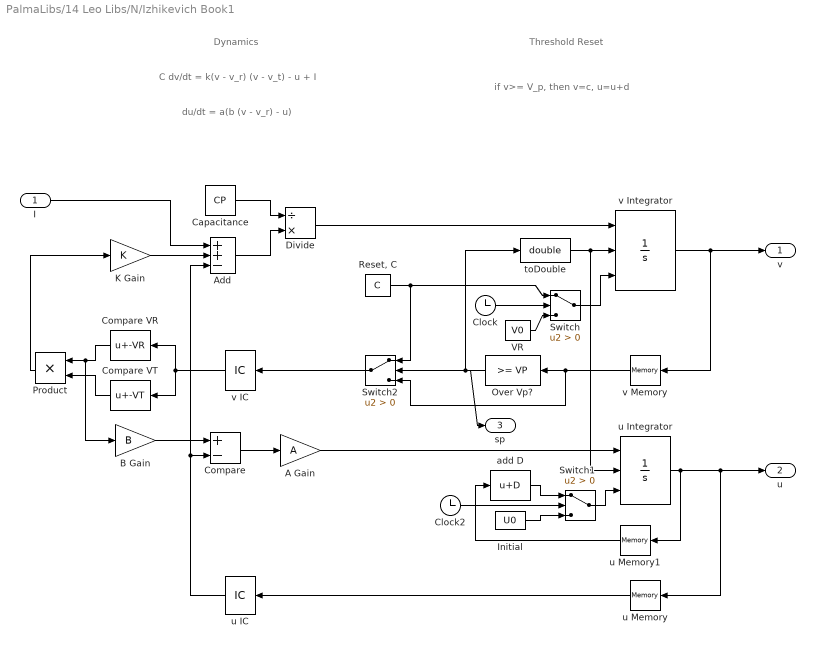
== system PalmaLibs/14 Leo Libs/N/Izhikevich Book1 ==
  note: C dv/dt = k(v - v_r) (v - v_t) - u + I
  note: du/dt = a(b (v - v_r) - u)
  note: if v>= V_p, then
      | v=c, u=u+d
  note: Dynamics
  note: Threshold Reset
  I : Inport
  " Initial" : Constant  Value=U0
  A Gain : Gain  Gain=A
  Add : Sum  Inputs=++-
  B Gain : Gain  Gain=B
  Capacitance : Constant  Value=CP
  Clock : Clock
  Clock2 : Clock
  Compare : Sum  Inputs=+-
  Compare VR : Bias  Bias=-VR
  Compare VT : Bias  Bias=-VT
  Divide : Product  Inputs=/*
  K Gain : Gain  Gain=K
  Over Vp? : simulink/Logic and Bit Operations/Compare To Constant  relop=>=  const=VP  OutDataTypeStr=boolean  ZeroCross=off
  Product : Product  RndMeth=Zero
  "Reset, C" : Constant  Value=C
  Switch : Switch  Criteria=u2 > Threshold  ZeroCross=off
  Switch1 : Switch  Criteria=u2 > Threshold  ZeroCross=off
  Switch2 : Switch  Criteria=u2 > Threshold  ZeroCross=off
  VR : Constant  Value=V0
  add D : Bias  Bias=D
  toDouble : DataTypeConversion  OutDataTypeStr=double
  u IC : InitialCondition  Value=U0
  u Integrator : Integrator  ExternalReset=rising  InitialConditionSource=external  ZeroCross=off
  u Memory : Memory
  u Memory1 : Memory
  v IC : InitialCondition  Value=V0
  v Integrator : Integrator  ExternalReset=rising  InitialConditionSource=external  InitialCondition=VR  ZeroCross=off
  v Memory : Memory
  v : Outport
  u : Outport  Port=2
  sp : Outport  Port=3
  wires:
  u Memory1/1 -> add D/1
  VR/1 -> Switch/3
  Capacitance/1 -> Divide/1
  Add/1 -> Divide/2
  toDouble/1 -> v Integrator/2, u Integrator/2
  v Integrator/1 -> v/1, v Memory/1
  K Gain/1 -> Add/2
  Compare VT/1 -> Product/2
  Compare VR/1 -> B Gain/1, Product/1
  I/1 -> Add/1
  Product/1 -> K Gain/1
  u Memory/1 -> u IC/1
  B Gain/1 -> Compare/1
  Compare/1 -> A Gain/1
  v IC/1 -> Compare VT/1, Compare VR/1
  u IC/1 -> Add/3, Compare/2
  Switch/1 -> v Integrator/3
  Clock/1 -> Switch/2
  "Reset, C"/1 -> Switch2/1, Switch/1
  u Integrator/1 -> u Memory1/1, u/1, u Memory/1
  Divide/1 -> v Integrator/1
  A Gain/1 -> u Integrator/1
  Clock2/1 -> Switch1/2
  Switch1/1 -> u Integrator/3
  add D/1 -> Switch1/1
  " Initial"/1 -> Switch1/3
  Switch2/1 -> v IC/1
  v Memory/1 -> Switch2/3, Over Vp?/1
  Over Vp?/1 -> sp/1, Switch2/2, toDouble/1

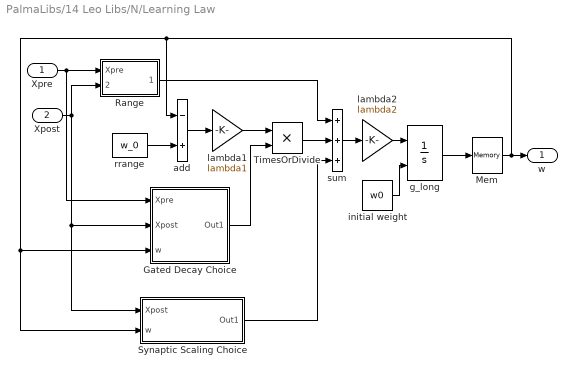
== system PalmaLibs/14 Leo Libs/N/Learning Law ==
  Xpre : Inport
  Xpost : Inport  Port=2
  Gated Decay Choice : Subsystem  BlockChoice=Gorch_Gating
      settings: AttributesFormatString=%<BlockChoice>  TemplateBlock=gated_decay_choice/Gated Decay Choice  MemberBlocks=Gorch_Gating,Oja_Gating,X_post,X_pre
  Mem : Memory
  Range : Subsystem  BlockChoice=Simple
      link override Gorch_range/range: Value=gorch_range
      settings: AttributesFormatString=%<BlockChoice>  TemplateBlock=range_choice/Range  MemberBlocks=Gorch_range,Simple
  Synaptic Scaling Choice : Subsystem  BlockChoice=None
      settings: AttributesFormatString=%<BlockChoice>  TemplateBlock=synaptic_scaling_choice/Synaptic Scaling Choice  MemberBlocks=None,Oja_stock
  TimesOrDivide : Product  Inputs=**
  add : Sum  Inputs=-+
  g_long : Integrator  InitialConditionSource=external  ZeroCross=off
  initial weight : Constant  Value=w0
  lambda1 : Gain  Gain=lambda1
  lambda2 : Gain  Gain=lambda2
  rrange : Constant  Value=w_0
  sum : Sum  Inputs=+++
  w : Outport
  wires:
  Xpre/1 -> Range/1(Xpre), Gated Decay Choice/1(Xpre)
  Xpost/1 -> Gated Decay Choice/2(Xpost), Synaptic Scaling Choice/1(Xpost), Range/2(Xpost)
  rrange/1 -> add/2
  Range/1(Out1) -> sum/1
  add/1 -> lambda1/1
  lambda1/1 -> TimesOrDivide/1
  TimesOrDivide/1 -> sum/2
  g_long/1 -> Mem/1
  initial weight/1 -> g_long/2
  Mem/1 -> Synaptic Scaling Choice/2(w), Gated Decay Choice/3(w), add/1, w/1
  Gated Decay Choice/1(Out1) -> TimesOrDivide/2
  lambda2/1 -> g_long/1
  sum/1 -> lambda2/1
  Synaptic Scaling Choice/1(Out1) -> sum/3

== system PalmaLibs/14 Leo Libs/XY3 Plot 1/New Axes ==
  Enable : EnablePort
  Axes : MATLABFcn  MATLABFcn=gca;
  Fig : MATLABFcn  MATLABFcn=figure(plotFig);
  h' : Outport
  wires:
  Axes/1 -> h'/1
  Fig/1 -> Axes/1

== system PalmaLibs/14 Leo Libs/XY3 Plot 1/Plot Update ==
  h : Inport
  X : Inport  Port=2
  Y : Inport  Port=3
  X2 : Inport  Port=4
  Y2 : Inport  Port=5
  X3 : Inport  Port=6
  Y3 : Inport  Port=7
  Enable : EnablePort
  L2 M-file S-Funct : M-S-Function  FunctionName=SPlot3
  h' : Outport
  wires:
  Y2/1 -> L2 M-file S-Funct/5
  X2/1 -> L2 M-file S-Funct/4
  h/1 -> L2 M-file S-Funct/1
  X/1 -> L2 M-file S-Funct/2
  Y/1 -> L2 M-file S-Funct/3
  L2 M-file S-Funct/1 -> h'/1
  X3/1 -> L2 M-file S-Funct/6
  Y3/1 -> L2 M-file S-Funct/7

== system PalmaLibs/14 Leo Libs/XY4 Plot 1/New Axes ==
  Enable : EnablePort
  Axes : MATLABFcn  MATLABFcn=gca;
  Fig : MATLABFcn  MATLABFcn=figure(plotFig);
  h' : Outport
  wires:
  Fig/1 -> Axes/1
  Axes/1 -> h'/1

== system PalmaLibs/14 Leo Libs/XY4 Plot 1/Plot Update ==
  h : Inport
  X : Inport  Port=2
  Y : Inport  Port=3
  X2 : Inport  Port=4
  Y2 : Inport  Port=5
  X3 : Inport  Port=6
  Y3 : Inport  Port=7
  X4 : Inport  Port=8
  Y4 : Inport  Port=9
  Enable : EnablePort
  L2 M-file S-Funct : M-S-Function  FunctionName=SPlot4
  h' : Outport
  wires:
  Y3/1 -> L2 M-file S-Funct/7
  X3/1 -> L2 M-file S-Funct/6
  L2 M-file S-Funct/1 -> h'/1
  Y/1 -> L2 M-file S-Funct/3
  X/1 -> L2 M-file S-Funct/2
  h/1 -> L2 M-file S-Funct/1
  X2/1 -> L2 M-file S-Funct/4
  Y2/1 -> L2 M-file S-Funct/5
  X4/1 -> L2 M-file S-Funct/8
  Y4/1 -> L2 M-file S-Funct/9

== system PalmaLibs/14 Leo Libs/bestfit Plot 1/New Axes ==
  Enable : EnablePort
  Axes : MATLABFcn  MATLABFcn=gca;
  Fig : MATLABFcn  MATLABFcn=figure(plotFig);
  h' : Outport
  wires:
  Axes/1 -> h'/1
  Fig/1 -> Axes/1

== system PalmaLibs/14 Leo Libs/bestfit Plot 1/Plot Update ==
  h : Inport
  X : Inport  Port=2
  Y : Inport  Port=3
  X2 : Inport  Port=4
  Y2 : Inport  Port=5
  X3 : Inport  Port=6
  Y3 : Inport  Port=7
  Enable : EnablePort
  L2 M-file S-Funct : M-S-Function  FunctionName=SPlot3d
  h' : Outport
  wires:
  Y2/1 -> L2 M-file S-Funct/5
  X2/1 -> L2 M-file S-Funct/4
  h/1 -> L2 M-file S-Funct/1
  X/1 -> L2 M-file S-Funct/2
  Y/1 -> L2 M-file S-Funct/3
  L2 M-file S-Funct/1 -> h'/1
  X3/1 -> L2 M-file S-Funct/6
  Y3/1 -> L2 M-file S-Funct/7

== system PalmaLibs/14 Leo Libs/Allan STD/Sum of Squares of Time Errors/x(t) ==
  note: x(t)
  note: nominal freq
  freq : Inport
  nom_freq : Inport  Port=2
  Divide1 : Product  Inputs=/*
  Multiply : Product  Inputs=**
  Subtract : Sum  Inputs=-+
  time : Clock
  x(t) : Outport
  wires:
  Subtract/1 -> x(t)/1
  Divide1/1 -> Subtract/2
  Multiply/1 -> Divide1/2
  time/1 -> Multiply/2, Subtract/1
  nom_freq/1 -> Divide1/1
  freq/1 -> Multiply/1

== system PalmaLibs/14 Leo Libs/Allan STD/Sum of Squares of Time Errors/x(t)1 ==
  note: nominal freq
  note: x(t)
  freq : Inport
  nom_freq : Inport  Port=2
  Divide1 : Product  Inputs=/*
  Multiply : Product  Inputs=**
  Subtract : Sum  Inputs=-+
  time : Clock
  x(t) : Outport
  wires:
  freq/1 -> Multiply/1
  nom_freq/1 -> Divide1/1
  time/1 -> Subtract/1, Multiply/2
  Multiply/1 -> Divide1/2
  Divide1/1 -> Subtract/2
  Subtract/1 -> x(t)/1

== system PalmaLibs/14 Leo Libs/Allan STD/Sum of Squares of Time Errors/x(t)2 ==
  note: x(t)
  note: nominal freq
  freq : Inport
  nom_freq : Inport  Port=2
  Divide1 : Product  Inputs=/*
  Multiply : Product  Inputs=**
  Subtract : Sum  Inputs=-+
  time : Clock
  x(t) : Outport
  wires:
  Subtract/1 -> x(t)/1
  Divide1/1 -> Subtract/2
  Multiply/1 -> Divide1/2
  time/1 -> Multiply/2, Subtract/1
  nom_freq/1 -> Divide1/1
  freq/1 -> Multiply/1

== system PalmaLibs/14 Leo Libs/N/Learning Law/Gated Decay Choice ==
  Xpre : Inport
  Xpost : Inport  Port=2
  w : Inport  Port=3
  Gorch_Gating : gated_decay_choice/Gorch_Gating
  Out1 : Outport
  wires:
  Xpre/1 -> Gorch_Gating/1
  Xpost/1 -> Gorch_Gating/2
  w/1 -> Gorch_Gating/3
  Gorch_Gating/1 -> Out1/1

== system PalmaLibs/14 Leo Libs/N/Learning Law/Range ==
  Xpre : Inport
  Xpost : Inport  Port=2
  Simple : range_choice/Simple  SystemSampleTime=-1
  Out1 : Outport
  wires:
  Xpre/1 -> Simple/1
  Xpost/1 -> Simple/2
  Simple/1 -> Out1/1

== system PalmaLibs/14 Leo Libs/N/Learning Law/Synaptic Scaling Choice ==
  Xpost : Inport
  w : Inport  Port=2
  None : synaptic_scaling_choice/None
  Out1 : Outport
  wires:
  Xpost/1 -> None/1
  w/1 -> None/2
  None/1 -> Out1/1
